simulink model "ejercicio2"  (R2020b)
settings: Solver=ode3  StartTime=0.0  StopTime=100  FixedStep=0.01  RelTol=1e-3
undefined symbols (not defined in the file or in its folder): DiscIntNeverNeededParam
libraries: simulink x1
settings Model: EnablePacing=on  Creator=patri  LastModifiedBy=patri

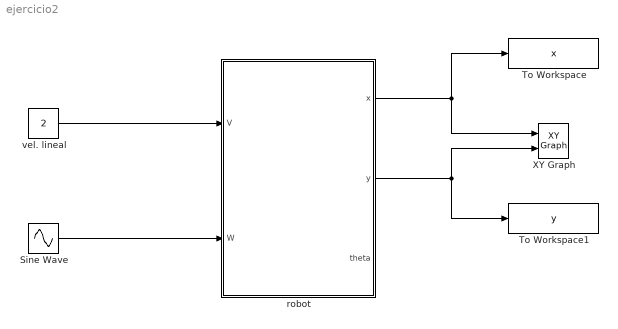
== system ejercicio2 ==
  Sine Wave : Sin  Amplitude=10  Frequency=10  SampleTime=0
  To Workspace : ToWorkspace  VariableName=x  SaveFormat=Timeseries  SampleTime=-1
  To Workspace1 : ToWorkspace  VariableName=y  SaveFormat=Timeseries  SampleTime=-1
  XY Graph : simulink/Sinks/XY Graph  xmin=-10  xmax=10  ymin=-10  ymax=10  st=-1
  robot : Subsystem
  vel. lineal : Constant  Value=2
  wires:
  vel. lineal/1 -> robot/1(V)
  Sine Wave/1 -> robot/2(W)
  robot/1(x) -> XY Graph/1, To Workspace/1
  robot/2(y) -> To Workspace1/1, XY Graph/2

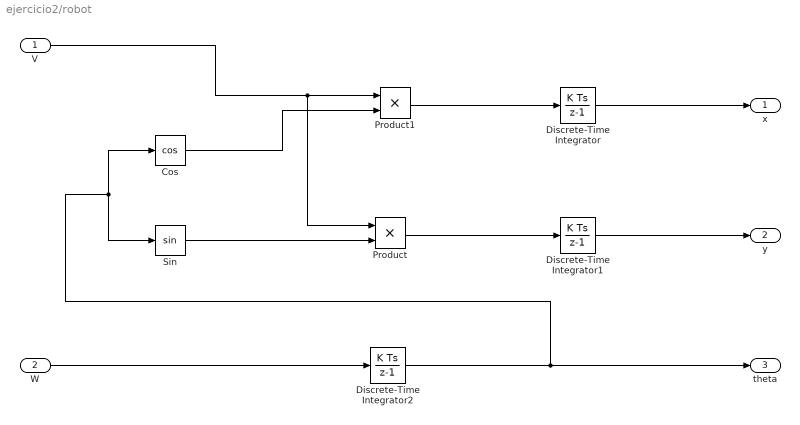
== system ejercicio2/robot ==
  V : Inport
  W : Inport  Port=2
  Cos : Trigonometry  Operator=cos
  Discrete-Time Integrator : DiscreteIntegrator  InitialCondition=-4  SampleTime=-1  ICPrevOutput=DiscIntNeverNeededParam  ICPrevScaledInput=DiscIntNeverNeededParam
  Discrete-Time Integrator1 : DiscreteIntegrator  InitialCondition=-4  SampleTime=-1  ICPrevOutput=DiscIntNeverNeededParam  ICPrevScaledInput=DiscIntNeverNeededParam
  Discrete-Time Integrator2 : DiscreteIntegrator  SampleTime=-1  ICPrevOutput=DiscIntNeverNeededParam  ICPrevScaledInput=DiscIntNeverNeededParam
  Product : Product
  Product1 : Product
  Sin : Trigonometry
  x : Outport
  y : Outport  Port=2
  theta : Outport  Port=3
  wires:
  Discrete-Time Integrator/1 -> x/1
  Discrete-Time Integrator1/1 -> y/1
  Product1/1 -> Discrete-Time Integrator/1
  Product/1 -> Discrete-Time Integrator1/1
  V/1 -> Product/1, Product1/1
  Cos/1 -> Product1/2
  Discrete-Time Integrator2/1 -> Sin/1, Cos/1, theta/1
  W/1 -> Discrete-Time Integrator2/1
  Sin/1 -> Product/2
